simulink model "CruiseControl"  (R2020a)
settings: Solver=VariableStepAuto  StartTime=0.0  StopTime=10.0  RelTol=1e-3
values from neighbouring files (symbols this model uses):
  b = 50.0    [CruseControlData.sldd]
  m = 1000.0    [CruseControlData.sldd]
settings Model: DataDictionary=CruseControlData.sldd  Creator=kasutav  LastModifiedBy=kasutav

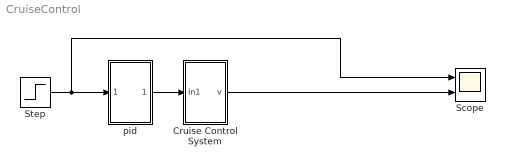
== system CruiseControl ==
  Cruise Control System : Subsystem
  Scope : Scope  NumInputPorts=2
  Step : Step  SampleTime=0
  pid : ModelReference  ModelNameDialog=Subsystem  ModelReferenceVersion=1.2
  wires:
  Step/1 -> pid/1, Scope/1
  Cruise Control System/1(v) -> Scope/2
  pid/1 -> Cruise Control System/1(In1)

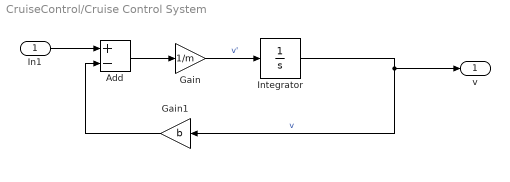
== system CruiseControl/Cruise Control System ==
  In1 : Inport
  Add : Sum  Inputs=+-
  Gain : Gain  Gain=1/m
  Gain1 : Gain  Gain=b
  Integrator : Integrator
  v : Outport
  wires:
  In1/1 -> Add/1
  Gain1/1 -> Add/2
  Add/1 -> Gain/1
  Gain/1 -> Integrator/1  "v'"
  Integrator/1 -> v/1, Gain1/1  "v"
